simulink model "half_car_model_active_suspension"  (R2023b)
settings: Solver=VariableStepAuto  StartTime=0.0  StopTime=20.0  RelTol=1e-3
values from neighbouring files (symbols this model uses):
  r0 = 0.1    [half_car_active_suspensions.m]
  x0 = [  2 ... (first row only)    [half_car_active_suspensions.m]
libraries: simulink x1
settings Model: Creator=alex2  LastModifiedBy=alex2

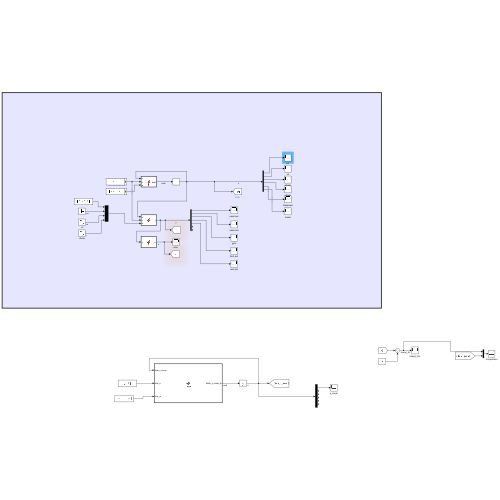
[thumbnail: Simulink's stored preview of the top-level diagram]
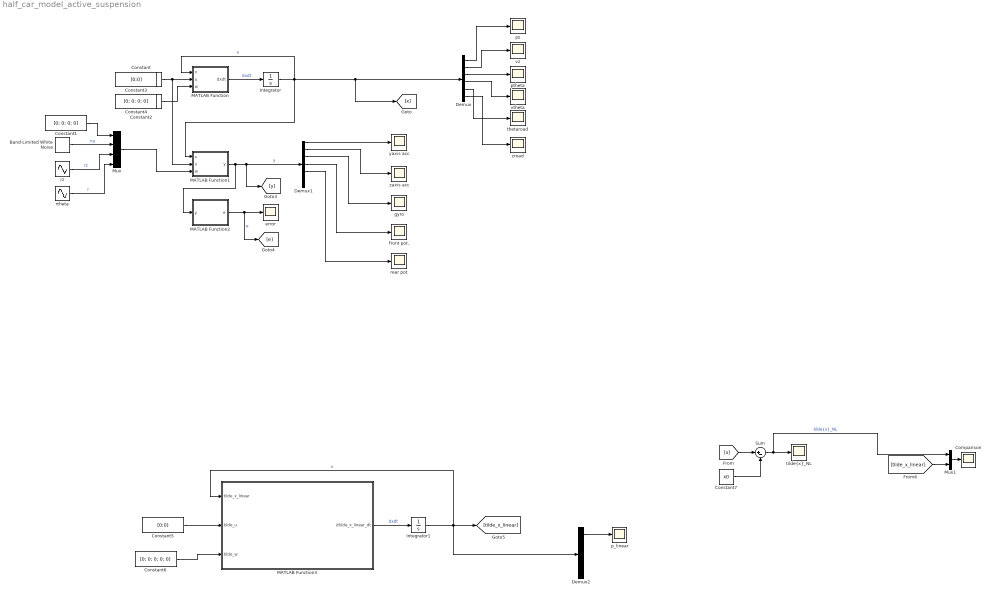
== system half_car_model_active_suspension ==
  Band-Limited White Noise : simulink/Sources/Band-Limited White Noise  Cov="1*[0.00001*1e-2; 0.00001*1e-2;  0.00001*1e-2; 0.00001*1e-2; 0.00001*1e-2]"  Ts=1e-2  seed=[23341; 31826; 11111; 81818; 00001]
  Comparison : Scope
  Constant : Constant  Value=[0;0]
  Constant1 : Constant  Value=[0; 0; 0; 0]
  Constant2 : Constant  Value=[0; 0; 0; 0]
  Constant3 : Constant  Value=[0;0]
  Constant4 : Constant  Value=[0; 0; 0; 0]
  Constant5 : Constant  Value=[0;0]
  Constant6 : Constant  Value=[0; 0; 0; 0; 0]
  Constant7 : Constant  Value=x0
  Demux : Demux  Outputs=6
  Demux1 : Demux  Outputs=7
  Demux2 : Demux  Outputs=6
  Integrator : Integrator  InitialCondition=x0
  Integrator1 : Integrator  InitialCondition=x0
  MATLAB Function : MATLAB Function  TreatAsAtomicUnit=on
  MATLAB Function1 : MATLAB Function  TreatAsAtomicUnit=on
  MATLAB Function2 : MATLAB Function  TreatAsAtomicUnit=on
  MATLAB Function3 : MATLAB Function  TreatAsAtomicUnit=on
  Mux : Mux
  Mux1 : Mux  Inputs=2
  Sum : Sum  Inputs=|+-
  "error " : Scope
  front pot. : Scope
  gyro : Scope
  p_linear : Scope
  ptheta : Scope
  pz : Scope
  rear pot : Scope
  rtheta : Sin  Amplitude=0  Bias=r0  Frequency=0  SampleTime=0
  rz : Sin  Amplitude=0  Bias=r0  Frequency=0  SampleTime=0
  thetaroad : Scope
  "tilde{x}_NL" : Scope
  vtheta : Scope
  vz : Scope
  yaxis acc : Scope
  zaxis acc : Scope
  zroad : Scope
  wires:
  MATLAB Function/1(dxdt) -> Integrator/1  "dxdt"
  Integrator/1 -> MATLAB Function1/1(x), [x], Demux/1, MATLAB Function/1(x)  "x"
  Constant/1 -> MATLAB Function1/2(u), MATLAB Function/2(u)
  Demux/1 -> pz/1
  Demux/2 -> vz/1
  Demux/3 -> ptheta/1
  Demux/4 -> vtheta/1
  Demux/5 -> thetaroad/1
  Demux/6 -> zroad/1
  Band-Limited White Noise/1 -> Mux/2  "nu"
  rz/1 -> Mux/3  "rz"
  Constant1/1 -> Mux/1
  Mux/1 -> MATLAB Function1/3(w)
  Constant2/1 -> MATLAB Function/3(w)
  MATLAB Function1/1(y) -> [y], Demux1/1, MATLAB Function2/1(y)  "y"
  Demux1/1 -> yaxis acc/1
  Demux1/2 -> zaxis acc/1
  Demux1/3 -> gyro/1
  Demux1/4 -> front pot./1
  Demux1/5 -> rear pot/1
  rtheta/1 -> Mux/4  "r"
  MATLAB Function2/1(e) -> [e], "error "/1  "e"
  Constant6/1 -> MATLAB Function3/3(tilde_w)
  Constant5/1 -> MATLAB Function3/2(tilde_u)
  MATLAB Function3/1(dtilde_x_linear_dt) -> Integrator1/1  "dxdt"
  Integrator1/1 -> Demux2/1, MATLAB Function3/1(tilde_x_linear), [tilde_x_linear]  "x"
  Sum/1 -> Mux1/1, "tilde{x}_NL"/1  "tilde{x}_NL"
  Constant7/1 -> Sum/2
  Mux1/1 -> Comparison/1
  [tilde_x_linear] -> Mux1/2
  [x] -> Sum/1
  Demux2/1 -> p_linear/1

== matlab function half_car_model_active_suspension/MATLAB Function ==
  data: x input; u input; dxdt output; w input
function dxdt = f(x,u,w)
%% parameters
m = 2;      % [kg] mass
k = 10;    % [N/m] spring stiffness
beta = 1;   % [N/(m/s)] damper coeff.
ell0 = 2;   % [m] 0-load lenght
g = 9.81;   % [m/s^2] gravity acceleration
df = 1;     % [m] distance between center of mass and front
dr = 1;     % [m] distance between center of mass and rear
J = 500;      % [kg*m^2] Moment of intertia
%% state
pz = x(1);        % [m] heigth of the center of mass of the car 
vz = x(2);        % [m/s] speed of the center of mass of the car 
ptheta = x(3);    % [Rad] pitch angle of the car 
vtheta = x(4);    % [Rad/s] angular speed of the car 
thetaroad = x(5); % [Rad]Road slope
zroad = x(6);     %[m]Road height 

%% disturbance
zgsecond = w(1);
alphag = w(2);
fwfront = w(3);
fwrear = w(4);

%todo: Vedere se servono due disturbi 

%% state evolution

s1 = pz+df*(sin(ptheta)-sin(thetaroad)); % height of front suspension
s3 = pz-dr*(sin(ptheta)-sin(thetaroad)); % height of rear suspension

s2 = vz+df*(vtheta*cos(ptheta)-zroad*cos(thetaroad)); % height speed of front suspension
s4 = vz-dr*(vtheta*cos(ptheta)-zroad*cos(thetaroad)); % height speed of rear suspension

lf = s1 + ell0;
lr = s3 + ell0;

%f2 = -g + (((-k*(s1-ell0)-beta*s2)+(-k*(s3-ell0)-beta*s4))+u(1))/m; %  con  ell0
%f4 = (df*(-k*(s1-ell0)-beta*s2)-dr*(-k*(s3-ell0)-beta*s4)+u(2)+fwfront*lf+fwrear*lr)/J; %

f2 = -g + (((-k*(s1)-beta*s2)+(-k*(s3)-beta*s4))+u(1))/m; %  senza ell0
f4 = (df*(-k*(s1)-beta*s2)-dr*(-k*(s3)-beta*s4)+u(2)+fwfront*lf+fwrear*lr)/J; %

dxdt = [vz;
        f2-zgsecond; 
        x(4);
        f4;
        x(6);
        alphag];
        




end

== matlab function half_car_model_active_suspension/MATLAB Function2 ==
  data: y input; e output
function e = E(y)

df = 1;     % [m] distance between center of mass and front
dr = 1;     % [m] distance between center of mass and rear


yy = y(1); % output of h block yaxisacc 
yz = y(2); % output of h block zaxisacc 
yg = y(3); % output of h block gyro
yf = y(4); % output of h block pot. front
yr = y(5); % output of h block pot. rear
 
%% ref
rz = y(6);
rtheta = y(7);

e = [
    (yf*dr+yr*df)/(dr+df)-rz; 
    asin((yy)/(sqrt(yy^2+yz^2)))-rtheta];
end

== matlab function half_car_model_active_suspension/MATLAB Function3 ==
  data: tilde_x_linear input; tilde_u input; dtilde_x_linear_dt output; tilde_w input
function dtilde_x_linear_dt = Linear(tilde_x_linear,tilde_u,tilde_w)



%% parameters

m = 2;      % [kg] mass
k = 10;    % [N/m] spring stiffness
beta = 1;   % [N/(m/s)] damper coeff.
ell0 = 1;   % [m] 0-load lenght
g = 9.81;   % [m/s^2] gravity acceleration
df = 1;     % [m] distance between center of mass and front
dr = 1;     % [m] distance between center of mass and rear
J = 500;      % [kg*m^2] Moment of intertia
%%matrix
delta0 = -m*g/(2*k);

A = [0, 1, 0, 0, 0, 0;
    -2*k/m, -2*beta/m, -k*(df-dr)/m, -beta*(df-dr)/m, k*(df-dr)/m, beta*(df-dr)/m;
    0, 0, 0, 1, 0, 0;
    -k*(df-dr)/J, -beta*(df-dr)/J, -k*(df^2+dr^2)/J, -beta*(df+dr)/J, k*(df^2+dr^2)/J, beta*(df+dr)/J;
    0, 0, 0, 0, 0, 1;
    0, 0, 0, 0, 0, 0];


B1 = [0,0;
     1/m, 0;
     0,0;
     0, 1/J;
     0,0;
     0,0];

B2 = [0,0,0,0,0;
      -1,0,0,0,0;
      0,0,0,0,0;
      0,0,(delta0+ell0)/J,(delta0+ell0)/J, 0;
      0,0,0,0,0;
      0,1,0,0,0];




%% state evolution
dtilde_x_linear_dt = A*tilde_x_linear+B1*tilde_u+B2*tilde_w;
end

== matlab function half_car_model_active_suspension/MATLAB Function1 ==
  data: x input; u input; y output; w input
function y = h(x, u, w)

%% parameters
m = 2;      % [kg] mass
k = 10;    % [N/m] spring stiffness
beta = 1;   % [N/(m/s)] damper coeff.
ell0 = 1;   % [m] 0-load lenght
g = 9.81;   % [m/s^2] gravity acceleration
df = 1;     % [m] distance between center of mass and front
dr = 1;     % [m] distance between center of mass and rear
J = 500;      % [kg*m^2] Moment of intertia

%% state
pz = x(1);        % [m] heigth of the center of mass of the car 
vz = x(2);        % [m/s] speed of the center of mass of the car 
ptheta = x(3);    % [Rad] pitch angle of the car 
vtheta = x(4);    % [Rad/s] angular speed of the car 
thetaroad = x(5); % [Rad]Road slope
zroad = x(6);     %[m]Road height 

%% state evolution

s1 = pz+df*(sin(ptheta)-sin(thetaroad)); % height of front suspension
s3 = pz-dr*(sin(ptheta)-sin(thetaroad)); % height of rear suspension

s2 = vz+df*(vtheta*cos(ptheta)-zroad*cos(thetaroad)); % height speed of front suspension
s4 = vz-dr*(vtheta*cos(ptheta)-zroad*cos(thetaroad)); % height speed of rear suspension

lf = s1 + ell0;
lr = s3 + ell0;

%f2 = -g + (((-k*(s1-ell0)-beta*s2)+(-k*(s3-ell0)-beta*s4))+u(1))/m; %  con ell0
%f4 = (df*(-k*(s1-ell0)-beta*s2)-dr*(-k*(s3-ell0)-beta*s4)+u(2)+fwfront*lf+fwrear*lr)/J; %

f2 = -g + (((-k*(s1)-beta*s2)+(-k*(s3)-beta*s4))+u(1))/m; % senza ell0
%f4 = (df*(-k*(s1)-beta*s2)-dr*(-k*(s3)-beta*s4)+u(2)+fwfront*lf+fwrear*lr)/J; %


zgsecond = w(1);
alphag = w(2);
fwfront = w(3);
fwrear = w(4);
nuy = w(5);
nuz = w(6);
nug = w(7);
nuf = w(8);
nur = w(9);

%% reference
rz = w(10);
rtheta=w(11);


%% output
y = [sin(x(3))*(f2 + g) + cos(x(3)) * ((fwrear + fwfront) / m)+nuy; 
     cos(x(3))*(f2 + g) - sin(x(3)) * ((fwrear + fwfront) / m)+nuz; %se facciamo cosi ci da in condizioni stazionarie Zaxisacc=9.81, se vogliamo il valore negativo mettere "-" davanti a coseno 
     x(4)+nug;
     s1+nuf;
     s3+nur;
     rz;
     rtheta];
end
